simulink model "T4_NonLinear_2_dof_Helicopter_Kalman"  (R2023a)
settings: Solver=ode4  StartTime=0.0  StopTime=inf  FixedStep=0.1  RelTol=1e-3
values from neighbouring files (symbols this model uses):
  Ac = [0,0,1,0 ... (first row only)    [Linerized_Parameters.m]
  B_p = 0.01    [Heli_Parameters.m]
  B_y = 0.08    [Heli_Parameters.m]
  Bc = [0,0 ... (first row only)    [Linerized_Parameters.m]
  Cc = [1,0,0,0 ... (first row only)    [Linerized_Parameters.m]
  g = 9.81    [Heli_Parameters.m]
  J_eqp = 0.0172    [Heli_Parameters.m]
  J_eqy = 0.0210    (= 0.021)    [Heli_Parameters.m]
  K_pp = 0.0556    [Heli_Parameters.m]
  K_py = 0.005    [Heli_Parameters.m]
  K_yp = 0.15    [Heli_Parameters.m]
  K_yy = 0.21084    [Heli_Parameters.m]
  l_cm = 0.015    [Heli_Parameters.m]
  m_heli = 0.479    [Heli_Parameters.m]
  p_op = pi/2    (= 1.57079632679)    [Linerized_Parameters.m]
  t_op = (-10*pi)/180    (= -0.174532925199)    [Linerized_Parameters.m]
  V_mp_op = (K_yy* m_heli*g*cos(t_op)*l_cm  )/((K_yy*K_pp-K_yp*K_py))    [Linerized_Parameters.m]
  V_my_op = (K_yp* V_mp_op)/K_yy    [Linerized_Parameters.m]
  wp_op = 0    [Linerized_Parameters.m]
  wt_op = 0    [Linerized_Parameters.m]
undefined symbols (not defined in the file or in its folder): L
libraries: realtime_pacer_lib x1
settings Model: Creator=aleho  LastModifiedBy=aleho

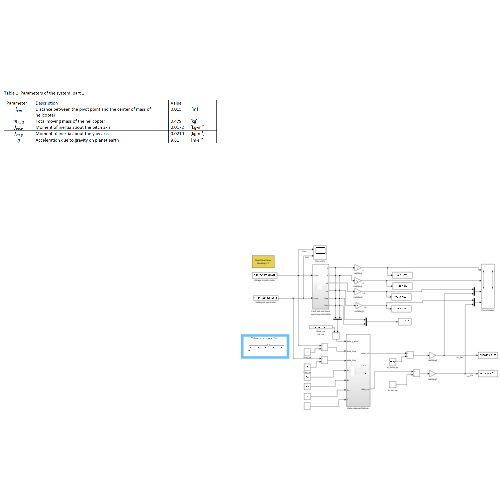
[thumbnail: Simulink's stored preview of the top-level diagram]
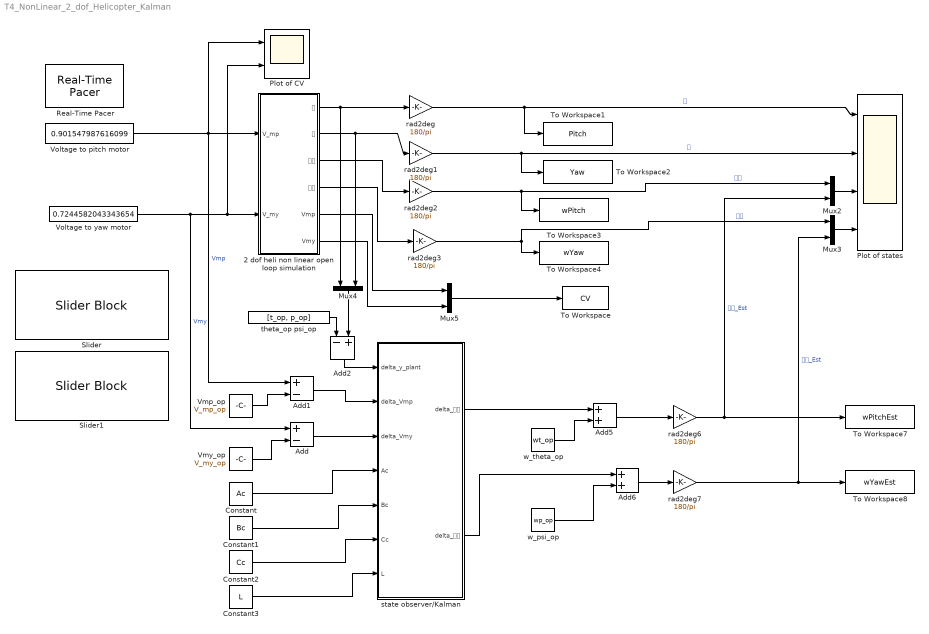
== system T4_NonLinear_2_dof_Helicopter_Kalman ==
  2 dof heli non linear open loop simulation : Subsystem
  Add : Sum  Inputs=+-
  Add1 : Sum  Inputs=+-
  Add2 : Sum  Inputs=-+
  Add5 : Sum
  Add6 : Sum
  Constant : Constant  Value=Ac
  Constant1 : Constant  Value=Bc
  Constant2 : Constant  Value=Cc
  Constant3 : Constant  Value=L
  Mux{2..5} (4 alike) : Mux  Inputs=2
  Plot of CV : Scope  NumInputPorts=2
  Plot of states : Scope  NumInputPorts=4
  Real-Time Pacer : realtime_pacer_lib/Real-Time Pacer  simTimePerRealTime=1
  Slider : SliderBlock  ScaleMax=1.4  TickInterval=1
  Slider1 : SliderBlock  ScaleMax=1.3  TickInterval=1
  To Workspace : ToWorkspace  VariableName=CV  SaveFormat=Timeseries  SampleTime=-1
  To Workspace1 : ToWorkspace  VariableName=Pitch  SaveFormat=Timeseries  SampleTime=-1
  To Workspace2 : ToWorkspace  VariableName=Yaw  SaveFormat=Timeseries  SampleTime=-1
  To Workspace3 : ToWorkspace  VariableName=wPitch  SaveFormat=Timeseries  SampleTime=-1
  To Workspace4 : ToWorkspace  VariableName=wYaw  SaveFormat=Timeseries  SampleTime=-1
  To Workspace7 : ToWorkspace  VariableName=wPitchEst  SaveFormat=Timeseries  SampleTime=-1
  To Workspace8 : ToWorkspace  VariableName=wYawEst  SaveFormat=Timeseries  SampleTime=-1
  Vmp_op : Constant  Value=V_mp_op
  Vmy_op : Constant  Value=V_my_op
  Voltage to pitch motor : Constant  Value=0.901547987616099
  Voltage to yaw motor : Constant  Value=0.7244582043343654
  rad2deg{,1..3,6..7} (6 alike) : Gain  Gain=180/pi
  state observer/Kalman : Subsystem
  theta_op psi_op : Constant  Value=[t_op, p_op]
  w_psi_op : Constant  Value=wp_op
  w_theta_op : Constant  Value=wt_op
  wires:
  Voltage to pitch motor/1 -> Add1/1, 2 dof heli non linear open loop simulation/1(V_mp), Plot of CV/1  "Vmp"
  Voltage to yaw motor/1 -> Plot of CV/2, 2 dof heli non linear open loop simulation/2(V_my), Add/1  "Vmy"
  2 dof heli non linear open loop simulation/1(𝜃) -> Mux4/1, rad2deg/1
  2 dof heli non linear open loop simulation/2(𝜓) -> Mux4/2, rad2deg1/1
  2 dof heli non linear open loop simulation/3(𝜔𝜃) -> rad2deg2/1
  2 dof heli non linear open loop simulation/4(𝜔𝜓) -> rad2deg3/1
  Vmy_op/1 -> Add/2
  Vmp_op/1 -> Add1/2
  theta_op psi_op/1 -> Add2/1
  Mux4/1 -> Add2/2
  Add2/1 -> state observer/Kalman/1(delta_y_plant)
  Add1/1 -> state observer/Kalman/2(delta_Vmp)
  rad2deg/1 -> To Workspace1/1, Plot of states/1  "𝜃"
  rad2deg1/1 -> Plot of states/2, To Workspace2/1  "𝜓"
  w_theta_op/1 -> Add5/2
  state observer/Kalman/1(delta_𝜔𝜃) -> Add5/1
  Mux2/1 -> Plot of states/3
  rad2deg2/1 -> Mux2/1, To Workspace3/1  "𝜔𝜃"
  Mux3/1 -> Plot of states/4
  rad2deg3/1 -> Mux3/1, To Workspace4/1  "𝜔𝜓"
  state observer/Kalman/2(delta_𝜔𝜓) -> Add6/1
  w_psi_op/1 -> Add6/2
  Add5/1 -> rad2deg6/1
  Add6/1 -> rad2deg7/1
  rad2deg6/1 -> To Workspace7/1, Mux2/2  "𝜔𝜃_Est"
  rad2deg7/1 -> To Workspace8/1, Mux3/2  "𝜔𝜓_Est"
  Add/1 -> state observer/Kalman/3(delta_Vmy)
  Constant1/1 -> state observer/Kalman/5(Bc)
  Constant2/1 -> state observer/Kalman/6(Cc)
  Constant/1 -> state observer/Kalman/4(Ac)
  Constant3/1 -> state observer/Kalman/7(L)
  Mux5/1 -> To Workspace/1
  2 dof heli non linear open loop simulation/5(Vmp) -> Mux5/1
  2 dof heli non linear open loop simulation/6(Vmy) -> Mux5/2

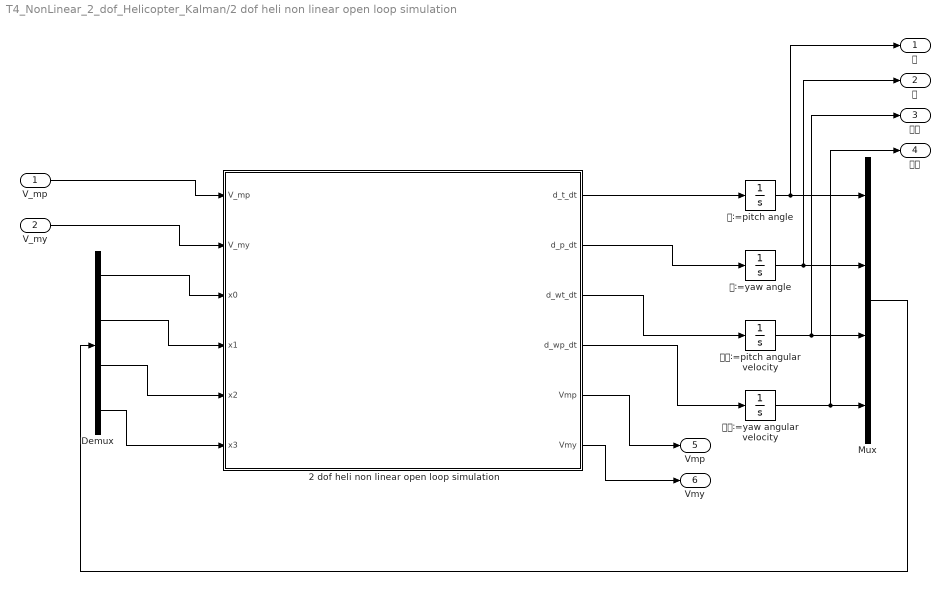
== system T4_NonLinear_2_dof_Helicopter_Kalman/2 dof heli non linear open loop simulation ==
  V_mp : Inport
  V_my : Inport  Port=2
  2 dof heli non linear open loop simulation : MATLAB Function  TreatAsAtomicUnit=on
  Demux : Demux
  Mux : Mux
  𝜃∶=pitch angle : Integrator  InitialCondition=-45*pi/180  LimitOutput=on  UpperSaturationLimit=45*pi/180  LowerSaturationLimit=-45*pi/180
  𝜓∶=yaw angle : Integrator  InitialCondition=pi/2  LimitOutput=on  UpperSaturationLimit=pi  LowerSaturationLimit=0
  𝜔𝜃∶=pitch angular velocity : Integrator  LimitOutput=on  UpperSaturationLimit=2  LowerSaturationLimit=-2
  𝜔𝜓∶=yaw angular velocity : Integrator  LimitOutput=on  UpperSaturationLimit=2  LowerSaturationLimit=-2
  𝜃 : Outport
  𝜓 : Outport  Port=2
  𝜔𝜃 : Outport  Port=3
  𝜔𝜓 : Outport  Port=4
  Vmp : Outport  Port=5
  Vmy : Outport  Port=6
  wires:
  V_mp/1 -> 2 dof heli non linear open loop simulation/1(V_mp)
  𝜔𝜃∶=pitch angular velocity/1 -> 𝜔𝜃/1, Mux/3
  Demux/4 -> 2 dof heli non linear open loop simulation/6(x3)
  𝜔𝜓∶=yaw angular velocity/1 -> 𝜔𝜓/1, Mux/4
  Mux/1 -> Demux/1
  𝜃∶=pitch angle/1 -> 𝜃/1, Mux/1
  𝜓∶=yaw angle/1 -> 𝜓/1, Mux/2
  2 dof heli non linear open loop simulation/1(d_t_dt) -> 𝜃∶=pitch angle/1
  V_my/1 -> 2 dof heli non linear open loop simulation/2(V_my)
  Demux/1 -> 2 dof heli non linear open loop simulation/3(x0)
  Demux/3 -> 2 dof heli non linear open loop simulation/5(x2)
  Demux/2 -> 2 dof heli non linear open loop simulation/4(x1)
  2 dof heli non linear open loop simulation/2(d_p_dt) -> 𝜓∶=yaw angle/1
  2 dof heli non linear open loop simulation/4(d_wp_dt) -> 𝜔𝜓∶=yaw angular velocity/1
  2 dof heli non linear open loop simulation/3(d_wt_dt) -> 𝜔𝜃∶=pitch angular velocity/1
  2 dof heli non linear open loop simulation/5(Vmp) -> Vmp/1
  2 dof heli non linear open loop simulation/6(Vmy) -> Vmy/1

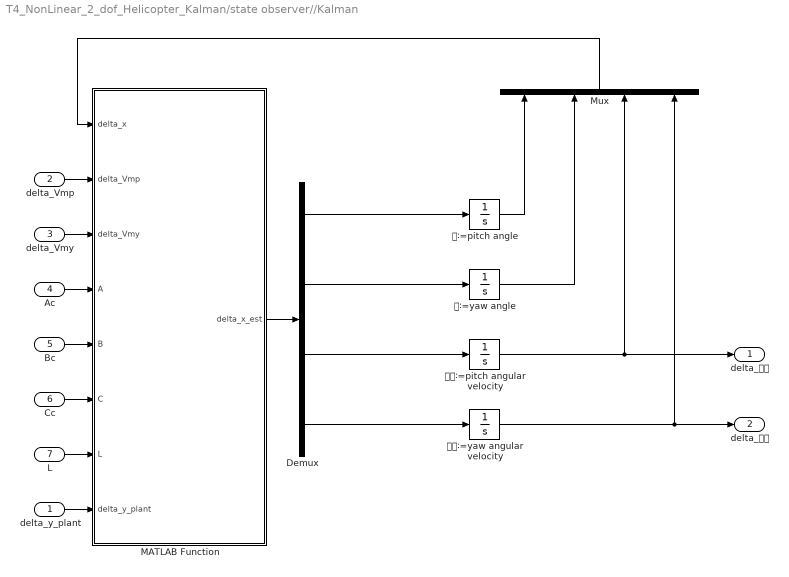
== system T4_NonLinear_2_dof_Helicopter_Kalman/state observer//Kalman ==
  delta_y_plant : Inport
  delta_Vmp : Inport  Port=2
  delta_Vmy : Inport  Port=3
  Ac : Inport  Port=4
  Bc : Inport  Port=5
  Cc : Inport  Port=6
  L : Inport  Port=7
  Demux : Demux
  MATLAB Function : MATLAB Function  TreatAsAtomicUnit=on
  Mux : Mux
  𝜃∶=pitch angle : Integrator  InitialCondition=-10*pi/180  LimitOutput=on  UpperSaturationLimit=45*pi/180  LowerSaturationLimit=-45*pi/180
  𝜓∶=yaw angle : Integrator  InitialCondition=pi/2  LimitOutput=on  UpperSaturationLimit=pi  LowerSaturationLimit=0
  𝜔𝜃∶=pitch angular velocity : Integrator  LimitOutput=on  UpperSaturationLimit=2  LowerSaturationLimit=-2
  𝜔𝜓∶=yaw angular velocity : Integrator  LimitOutput=on  UpperSaturationLimit=2  LowerSaturationLimit=-2
  delta_𝜔𝜃 : Outport
  delta_𝜔𝜓 : Outport  Port=2
  wires:
  delta_Vmp/1 -> MATLAB Function/2(delta_Vmp)
  delta_Vmy/1 -> MATLAB Function/3(delta_Vmy)
  MATLAB Function/1(delta_x_est) -> Demux/1
  Demux/1 -> 𝜃∶=pitch angle/1
  Demux/2 -> 𝜓∶=yaw angle/1
  Demux/3 -> 𝜔𝜃∶=pitch angular velocity/1
  Demux/4 -> 𝜔𝜓∶=yaw angular velocity/1
  𝜔𝜓∶=yaw angular velocity/1 -> Mux/4, delta_𝜔𝜓/1
  𝜔𝜃∶=pitch angular velocity/1 -> Mux/3, delta_𝜔𝜃/1
  𝜃∶=pitch angle/1 -> Mux/1
  𝜓∶=yaw angle/1 -> Mux/2
  Mux/1 -> MATLAB Function/1(delta_x)
  Ac/1 -> MATLAB Function/4(A)
  Bc/1 -> MATLAB Function/5(B)
  Cc/1 -> MATLAB Function/6(C)
  L/1 -> MATLAB Function/7(L)
  delta_y_plant/1 -> MATLAB Function/8(delta_y_plant)

== matlab function T4_NonLinear_2_dof_Helicopter_Kalman/state observer//Kalman/MATLAB Function ==
  data: delta_x input; delta_Vmp input; delta_Vmy input; A input; B input; C input; L input; delta_y_plant input; delta_x_est output
function delta_x_est  = linear_observer(delta_x, delta_Vmp, delta_Vmy, A,B,C,L, delta_y_plant)

y_est = C*delta_x;
delta_x_est = A*delta_x+B*[delta_Vmp;delta_Vmy] + L*(delta_y_plant-y_est); % L = Kf(Kalman gain)

== matlab function T4_NonLinear_2_dof_Helicopter_Kalman/2 dof heli non linear open loop simulation/2 dof heli non linear open loop simulation ==
  data: V_mp input; V_my input; d_t_dt output; d_p_dt output; d_wt_dt output; d_wp_dt output; x0 input; x1 input; x2 input; x3 input; l_cm parameter; m_heli parameter; J_eqp parameter; J_eqy parameter; g parameter; K_pp parameter; K_yy parameter; K_py parameter; K_yp parameter; B_p parameter; B_y parameter; Vmp output; Vmy output
function [d_t_dt,d_p_dt,d_wt_dt,d_wp_dt, Vmp, Vmy] =  heli_2_dof_ODE_eqs(V_mp,V_my,x0,x1,x2,x3, l_cm, m_heli, ...
    J_eqp, J_eqy, g, K_pp, K_yy, K_py, K_yp, B_p, B_y)
% States
t = x0;    % pitch angle ( theta )
p = x1;    % yaw angle ( psi )
wt = x2;   % pitch angular velocity ( Omega theta )
wp = x3;   % yaw angular velocity ( Omega psi )

Vmp = V_mp;
Vmy = V_my;

% ODEs

% pitch angle
d_t_dt = wt;

% yaw angle
d_p_dt = wp;

% pitch angular velocity
d_wt_dt = ((K_pp*V_mp)/(J_eqp+m_heli*l_cm^2)) - ((K_py*V_my)/(J_eqp+m_heli*l_cm^2))...
    - ((B_p*wt+m_heli*wp^2*sin(t)*l_cm^2*cos(t)+m_heli*g*cos(t)*l_cm) / (J_eqp+m_heli*l_cm^2));

% yaw angular velocity
d_wp_dt = ((K_yp*V_mp)/(J_eqy+m_heli*cos(t)^2*l_cm^2)) -...
    ((K_yy*V_my)/(J_eqy+m_heli*cos(t)^2*l_cm^2)) +...
    ((2*m_heli*wp*sin(t)*l_cm^2*cos(t)*wt)/(J_eqy+m_heli*cos(t)^2*l_cm^2))...
    - ((B_y*wp)/(J_eqy+m_heli*cos(t)^2*l_cm^2));
